simulink model "cancello_2022b"  (R2024a)
settings: Solver=FixedStepAuto  StartTime=0.0  StopTime=120  FixedStep=0.1  RelTol=1e-3
settings Model: NumberOfSteps=2  Creator=vcarletti  LastModifiedBy=franc
settings OptimizationCC: DefaultParameterBehavior=Inlined  UseDivisionForNetSlopeComputation=on  GainParamInheritBuiltInType=on  UseFloatMulNetSlope=on  InlineInvariantSignals=on  PassReuseOutputArgsAs=Individual arguments  ZeroExternalMemoryAtStartup=off  ZeroInternalMemoryAtStartup=off  NoFixptDivByZeroProtection=on  EfficientFloat2IntCast=on  LifeSpan=1  OptimizeBlockOrder=speed  DifferentSizesBufferReuse=on  EfficientTunableParamExpr=on
settings DebuggingCC: ParameterTunabilityLossMsg=error
settings HardwareCC: ProdBitPerPointer=32  ProdBitPerSizeT=32  ProdBitPerPtrDiffT=32  ProdLargestAtomicInteger=Long  ProdLargestAtomicFloat=Double  ProdWordSize=32  ProdLongLongMode=on  ProdHWDeviceType=ARM Compatible->ARM Cortex-M
settings SFSimCC: MATLABDynamicMemAlloc=off
settings RTWCC: Description=Embedded Coder  SystemTargetFile=ert.tlc  TemplateMakefile=ert_default_tmf  GenerateReport=on  LaunchReport=on
settings CodeAppCC: ForceParamTrailComments=on  IgnoreCustomStorageClasses=off  OperatorAnnotations=on  SimulinkDataObjDesc=on  SFDataObjDesc=on  CustomSymbolStrGlobalVar=rt$N$M  CustomSymbolStrType=$N$M  CustomSymbolStrFcn=$N$M$F  CustomSymbolStrMacro=$N$M  InsertBlockDesc=on
settings ERTTargetCC: TargetLangStandard=C99 (ISO)  GenerateSampleERTMain=on  IncludeMdlTerminateFcn=off  CombineSignalStateStructs=on  SupportAbsoluteTime=off  PurelyIntegerCode=on  SupportComplex=off  SupportNonInlinedSFcns=on  InlinedParameterPlacement=NonHierarchical  ERTCustomFileTemplate=example_file_process.tlc  ERTFilePackagingFormat=CompactWithDataFile
settings ConfigComp: CovEnable=on  RecordCoverage=on  CovSaveSingleToWorkspaceVar=on  CovOutputDir=/MATLAB Drive/SistemiEmb2/  CovDataFileName=GeneralCoverage  CovModelRefEnable=on

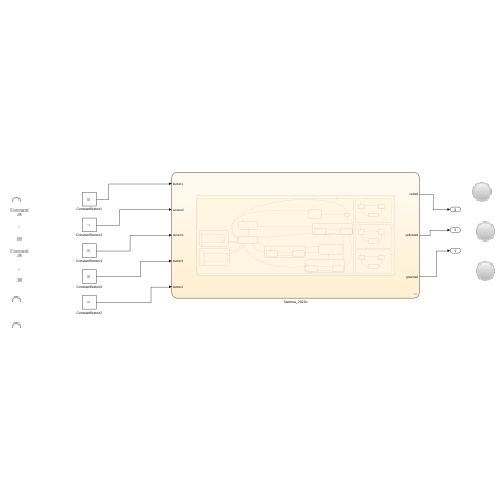
[thumbnail: Simulink's stored preview of the top-level diagram]
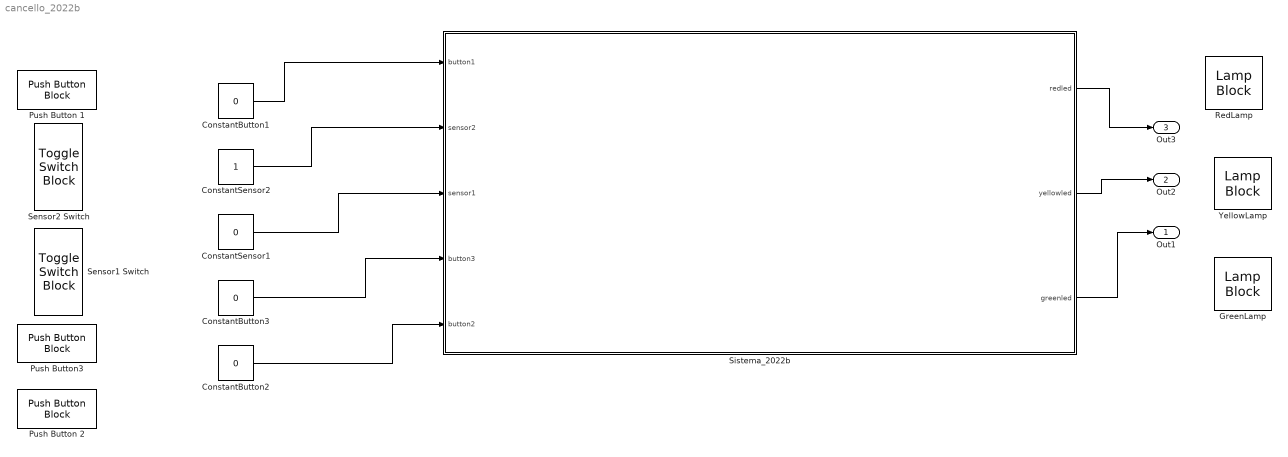
== system cancello_2022b ==
  ConstantButton1 : Constant  Value=0  OutDataTypeStr=boolean
  ConstantButton2 : Constant  Value=0  OutDataTypeStr=boolean
  ConstantButton3 : Constant  Value=0  OutDataTypeStr=boolean
  ConstantSensor1 : Constant  Value=0  OutDataTypeStr=boolean
  ConstantSensor2 : Constant  OutDataTypeStr=boolean
  GreenLamp : LampBlock  LabelPosition=Hide
  Push Button 1 : PushButtonBlock  ButtonText=Button1  OffValue=0.000000
  Push Button 2 : PushButtonBlock  ButtonText=Button2  OffValue=0.000000
  Push Button3 : PushButtonBlock  ButtonText=Button3  OffValue=0.000000
  RedLamp : LampBlock  LabelPosition=Hide
  Sensor1 Switch : ToggleSwitchBlock
      settings: Values={{'Off', 'On'}, [0 1]}
  Sensor2 Switch : ToggleSwitchBlock
      settings: Values={{'Off', 'On'}, [0 1]}
  Sistema_2022b : Stateflow chart  TreatAsAtomicUnit=on
  YellowLamp : LampBlock  LabelPosition=Hide
  Out1 : Outport
  Out2 : Outport  Port=2
  Out3 : Outport  Port=3
  wires:
  Sistema_2022b/3(greenled) -> Out1/1
  Sistema_2022b/2(yellowled) -> Out2/1
  Sistema_2022b/1(redled) -> Out3/1
  ConstantButton1/1 -> Sistema_2022b/1(button1)
  ConstantSensor2/1 -> Sistema_2022b/2(sensor2)
  ConstantSensor1/1 -> Sistema_2022b/3(sensor1)
  ConstantButton3/1 -> Sistema_2022b/4(button3)
  ConstantButton2/1 -> Sistema_2022b/5(button2)

== stateflow chart cancello_2022b/Sistema_2022b ==
  settings: updateMethod=DISCRETE  sampleTime=0.1
  state LOGIC
    state CANCELLO [parallel]
      settings: executionOrder=1
      state STATO_ALLARME
        en:
        redled = ON;
        exit:
        redled=OFF;
      state ERRORE
      state AVVIO
        en:
        tempo_di_lavoro=10;
        tempo_di_chiusura=10;
      state CHIUSURA
        state YELLOW_spento
          en:
          redled = OFF;
          yellowled=OFF;
          greenled=OFF;
        state YELLOW_acceso
          en:
          yellowled=ON;
          exit:
          yellowled=OFF;
        (default) -> LOGIC.CANCELLO.CHIUSURA.YELLOW_spento
        LOGIC.CANCELLO.CHIUSURA.YELLOW_spento -> LOGIC.CANCELLO.CHIUSURA.YELLOW_acceso : [after(toggling_period_yellow, sec)]
        LOGIC.CANCELLO.CHIUSURA.YELLOW_acceso -> LOGIC.CANCELLO.CHIUSURA.YELLOW_spento : [after(toggling_period_yellow, sec)]
      state TEMPO_DI_LAVORO
        (default) -> (junction 211)
        (junction 211) -> (junction 212) [order 1] : [tempo_di_lavoro==120]
        (junction 211) -> (junction 209) [order 2] : {tempo_di_lavoro=tempo_di_lavoro+10;}
        (junction 212) -> (junction 216) : {tempo_di_lavoro=10;}
        (junction 216) -> (junction 209)
        (junction 209) -> (junction 218)
      state CHIUSO
        en:
        redled = OFF;
        yellowled=OFF;
        greenled=OFF;
      state APERTO
        en:
        redled = ON;
        yellowled=ON;
        greenled=ON;
        exit:
        redled = OFF;
        yellowled=OFF;
        greenled=OFF;
      state RIGETTO_RICHIESTA
        state GREEN_spento
          en:
          redled = OFF;
          yellowled=OFF;
          greenled=OFF;
        state GREEN_acceso
          en:
          greenled=ON;
          exit:
          greenled=OFF;
        (default) -> GREEN_spento
        GREEN_spento -> GREEN_acceso : [after(toggling_period_green, sec)]
        GREEN_acceso -> GREEN_spento : [after(toggling_period_green, sec)]
      state TEMPO_DI_CHIUSURA
        (default) -> (junction 124)
        (junction 124) -> (junction 121) [order 1] : [tempo_di_chiusura==120]
        (junction 124) -> (junction 153) [order 2] : {tempo_di_chiusura=tempo_di_chiusura+10;}
        (junction 121) -> (junction 152) : {tempo_di_chiusura=10;}
        (junction 152) -> (junction 153)
        (junction 153) -> (junction 158)
      state APERTURA
        state YELLOW_spento
          en:
          redled = OFF;
          yellowled=OFF;
          greenled=OFF;
        state YELLOW_acceso
          en:
          yellowled=ON;
          exit:
          yellowled=OFF;
        (default) -> LOGIC.CANCELLO.APERTURA.YELLOW_spento
        LOGIC.CANCELLO.APERTURA.YELLOW_spento -> LOGIC.CANCELLO.APERTURA.YELLOW_acceso : [after(toggling_period_yellow, sec)]
        LOGIC.CANCELLO.APERTURA.YELLOW_acceso -> LOGIC.CANCELLO.APERTURA.YELLOW_spento : [after(toggling_period_yellow, sec)]
      ERRORE -> CHIUSO [order 2] : [sensor2==IS_PRESENT]
      STATO_ALLARME -> CHIUSO : [sensor2==IS_PRESENT]
      ERRORE -> STATO_ALLARME [order 1] : [sensor2~=IS_PRESENT && after(TIMER_ALLARME, sec)]
      CHIUSURA -> ERRORE [order 3] : [after(tempo_di_lavoro, sec) && sensor2~=IS_PRESENT]
      (default) -> AVVIO
      AVVIO -> CHIUSURA [order 2] : [sensor2~=IS_PRESENT]
      AVVIO -> CHIUSO [order 1] : [sensor2==IS_PRESENT]
      CHIUSURA -> CHIUSO [order 2] : [sensor2==IS_PRESENT]
      APERTO -> CHIUSURA [order 1] : [sensor1~=IS_PRESENT && (buttonpressed1 || after(tempo_di_chiusura,sec))]
      CHIUSURA -> APERTURA [order 1] : [buttonpressed1 || sensor1==IS_PRESENT]
      APERTURA -> CHIUSURA [order 1] : [buttonpressed1]
      CHIUSO -> TEMPO_DI_LAVORO [order 3] : [buttonpressed3]
      TEMPO_DI_LAVORO -> CHIUSO
      RIGETTO_RICHIESTA -> CHIUSO [order 1] : [sensor2==IS_PRESENT && (after(TIMER_RIGETTO, sec) || sensor1~=IS_PRESENT)]
      CHIUSO -> TEMPO_DI_CHIUSURA [order 4] : [buttonpressed2]
      TEMPO_DI_CHIUSURA -> CHIUSO
      CHIUSO -> APERTURA [order 1] : [buttonpressed1 && sensor1 ~= IS_PRESENT]
      CHIUSO -> RIGETTO_RICHIESTA [order 2] : [buttonpressed1 && sensor1==IS_PRESENT]
      RIGETTO_RICHIESTA -> APERTO [order 2] : [sensor2~=IS_PRESENT && (after(TIMER_RIGETTO, sec) || sensor1~=IS_PRESENT)]
      APERTO -> RIGETTO_RICHIESTA [order 2] : [buttonpressed1 && sensor1==IS_PRESENT]
      APERTURA -> APERTO [order 2] : [after(tempo_di_lavoro, sec)]
    state BUTTON1 [parallel]
      settings: executionOrder=2
      state RELEASED
      state PRESSED
      state LONGPRESSED
        send(buttonpressed1)
      (default) -> LOGIC.BUTTON1.RELEASED
      LOGIC.BUTTON1.RELEASED -> LOGIC.BUTTON1.PRESSED : [button1==ON]
      LOGIC.BUTTON1.LONGPRESSED -> LOGIC.BUTTON1.RELEASED : [button1== OFF]
      LOGIC.BUTTON1.PRESSED -> LOGIC.BUTTON1.LONGPRESSED : [button1== OFF]
    state BUTTON2 [parallel]
      settings: executionOrder=3
      state RELEASED
      state PRESSED
      state LONGPRESSED
        send(buttonpressed2)
      (default) -> LOGIC.BUTTON2.RELEASED
      LOGIC.BUTTON2.RELEASED -> LOGIC.BUTTON2.PRESSED : [button2==ON]
      LOGIC.BUTTON2.LONGPRESSED -> LOGIC.BUTTON2.RELEASED : [button2== OFF]
      LOGIC.BUTTON2.PRESSED -> LOGIC.BUTTON2.LONGPRESSED : [button2== OFF]
    state BUTTON3 [parallel]
      settings: executionOrder=4
      state RELEASED
      state PRESSED
      state LONGPRESSED
        send(buttonpressed3)
      (default) -> LOGIC.BUTTON3.RELEASED
      LOGIC.BUTTON3.RELEASED -> LOGIC.BUTTON3.PRESSED : [button3==ON]
      LOGIC.BUTTON3.LONGPRESSED -> LOGIC.BUTTON3.RELEASED : [button3== OFF]
      LOGIC.BUTTON3.PRESSED -> LOGIC.BUTTON3.LONGPRESSED : [button3== OFF]
    (default) -> CANCELLO [order 1]
    (default) -> BUTTON1 [order 2]
    (default) -> BUTTON2 [order 4]
    (default) -> BUTTON3 [order 3]
  data: button1 input boolean; redled output boolean; yellowled output boolean; OFF constant boolean =0; ON constant boolean =1; tempo_di_chiusura local int16; tempo_di_lavoro local int16; toggling_period_yellow constant int16 =2; sensor2 input boolean; sensor1 input boolean; TIMER_ALLARME constant int16 =10; TIMER_RIGETTO constant int16 =30; greenled output boolean; toggling_period_green constant int16 =1; button3 input boolean; button2 input boolean; IS_PRESENT constant boolean =true
  events: buttonpressed1 local FUNCTION_CALL_EVENT; buttonpressed2 local FUNCTION_CALL_EVENT; buttonpressed3 local FUNCTION_CALL_EVENT
